simulink model "ClosedLoop_Test"  (R2023b)
settings: Solver=VariableStepAuto  StartTime=0.0  StopTime=10.0  RelTol=1e-3
libraries: cstblocks x7
settings Model: Creator=Albertlakers  LastModifiedBy=Albertlakers

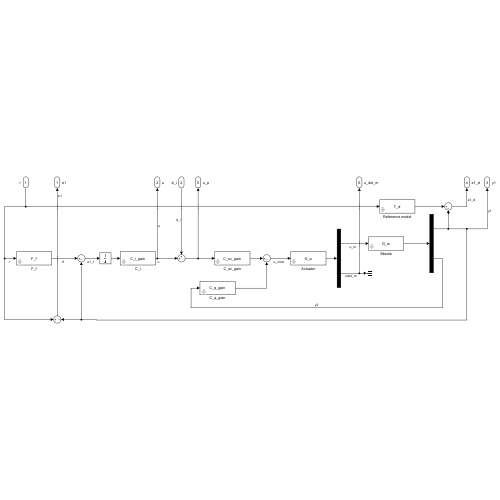
[thumbnail: Simulink's stored preview of the top-level diagram]
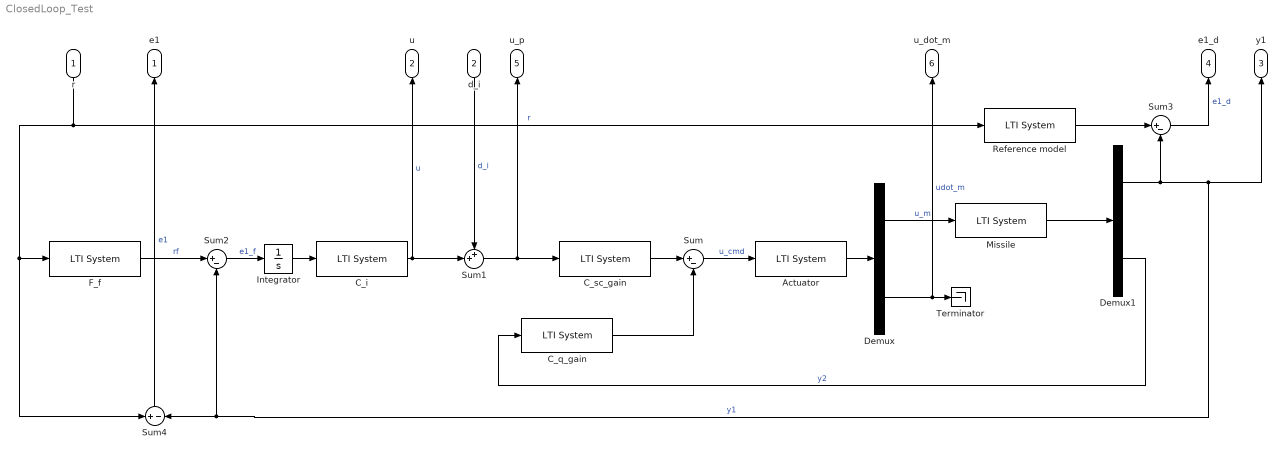
== system ClosedLoop_Test ==
  r : Inport
  d_i : Inport  Port=2
  Actuator : cstblocks/LTI System  sys=G_a  IC=[]  PadeOrder=0
  C_i : cstblocks/LTI System  sys=C_i_gain  IC=[]  PadeOrder=0
  C_q_gain : cstblocks/LTI System  sys=C_q_gain  IC=[]  PadeOrder=0
  C_sc_gain : cstblocks/LTI System  sys=C_sc_gain  IC=[]  PadeOrder=0
  Demux : Demux  Outputs=2
  Demux1 : Demux  Outputs=2
  F_f : cstblocks/LTI System  sys=F_f  IC=[]  PadeOrder=0
  Integrator : Integrator
  Missile : cstblocks/LTI System  sys=G_m  IC=[]  PadeOrder=0
  Reference model : cstblocks/LTI System  sys=T_d  IC=[]  PadeOrder=0
  Sum : Sum  Inputs=|+-
  Sum1 : Sum  Inputs=++|
  Sum2 : Sum  Inputs=|+-
  Sum3 : Sum  Inputs=|+-
  Sum4 : Sum  Inputs=+|-
  Terminator : Terminator
  e1 : Outport
  u : Outport  Port=2
  y1 : Outport  Port=3
  e1_d : Outport  Port=4
  u_p : Outport  Port=5
  u_dot_m : Outport  Port=6
  wires:
  Integrator/1 -> C_i/1
  Sum/1 -> Actuator/1  "u_cmd"
  Actuator/1 -> Demux/1
  Demux1/1 -> Sum4/2, Sum2/2, y1/1, Sum3/2  "y1"
  C_sc_gain/1 -> Sum/1
  Demux1/2 -> C_q_gain/1  "y2"
  C_q_gain/1 -> Sum/2
  Demux/2 -> u_dot_m/1, Terminator/1  "udot_m"
  Demux/1 -> Missile/1  "u_m"
  Missile/1 -> Demux1/1
  Sum1/1 -> u_p/1, C_sc_gain/1
  C_i/1 -> Sum1/2, u/1  "u"
  Sum2/1 -> Integrator/1  "e1_f"
  F_f/1 -> Sum2/1  "rf"
  Reference model/1 -> Sum3/1
  Sum3/1 -> e1_d/1  "e1_d"
  Sum4/1 -> e1/1  "e1"
  r/1 -> Reference model/1, F_f/1, Sum4/1  "r"
  d_i/1 -> Sum1/1  "d_i"
